simulink model "morrison"  (Simulink 7.8)
settings: Solver=ode45  StartTime=0.0  StopTime=2000.0  RelTol=1e-3
undefined symbols (not defined in the file or in its folder): inRate, shift
libraries: WaveformsLib x4, simulink x2
settings Model: Creator=Leo  LastModifiedBy=Leo

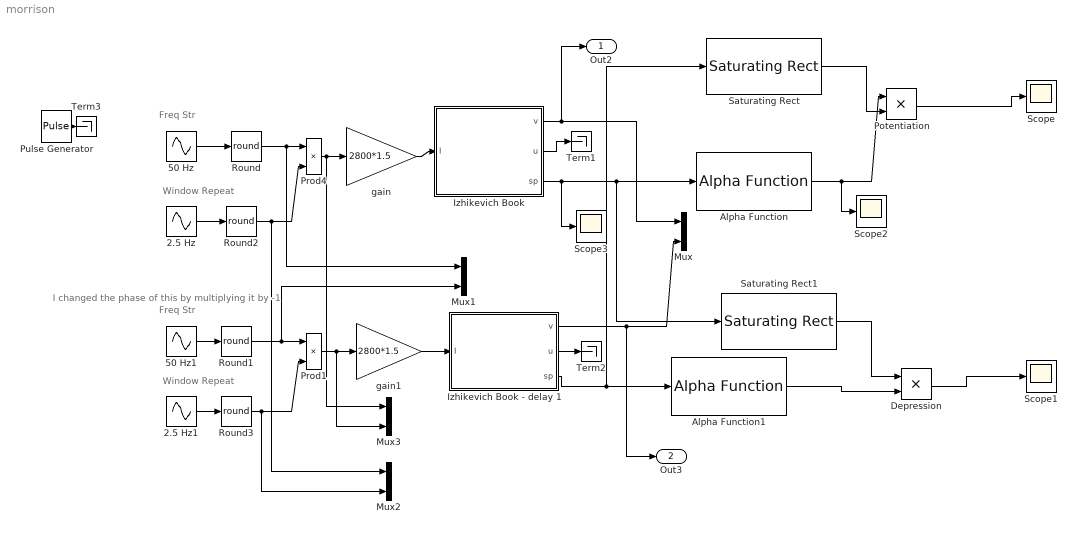
== system morrison ==
  note: Window Repeat
  note: Freq Str
  note: Window Repeat
  note: Freq Str
  note: I changed the phase of this by multiplying it by -1
  2.5 Hz : Sin  Amplitude=0.5  Bias=0.25  Frequency=2.5*2*pi/1000  Phase=pi  SampleTime=0
  2.5 Hz1 : Sin  Amplitude=0.5  Bias=0.25  Frequency=2.5*2*pi/1000  Phase=pi+shift*100/(2*pi*1000)  SampleTime=0
  50 Hz : Sin  Amplitude=0.5  Bias=inRate/20000  Frequency=inRate*2*pi/1000  Phase=-0*100/(2*pi*inRate)  SampleTime=0
  50 Hz1 : Sin  Amplitude=0.5  Bias=inRate/20000  Frequency=(inRate*2*pi)/1000  Phase=-shift*100/(2*pi*inRate)  SampleTime=0
  Alpha Function : WaveformsLib/Alpha Function  tauDecay=2  onsetStr=1
  Alpha Function1 : WaveformsLib/Alpha Function  tauDecay=2  onsetStr=1
  Depression : Product  RndMeth=Zero
  Izhikevich Book : Subsystem  AncestorBlock=CompartmentsLib/Izhikevich Book  mask{settings=UserDefined, A=0.03, B=-2, C=-50, D=100, CP=100, K=0.7, VR=-60, VT=-40, VP=35, V0=-60, U0=0}
      mask prompts: settings "Parameter Settings"; A "a, recovery u time constant"; B "b, dynamics parameter"; C "c,  reset value v"; D "d, reset shift u"; CP "Cp, capacitance"; VR "Vr, voltage rest"; VT "Vt, voltage threshold"; VP "Vpeak, voltage peak reset"; V0 "V0, initial v value"; U0 "U0, initial u value"
      mask help:
      | Model from Eugene Izhikevich's book "Dynamical Systems in Neuroscience"
      |     (Equations 8.5 & 8.6 on page 273)
      | 9 Paramters are reducable to 4-parameter model.
      |
      | Simulink Model Design: Jesse Palma
      mask Help:
      | Model from Eugene Izhikevich's book
      | <a href=http://www.izhikevich.org/publications/dsn/index.htm>"Dynamical Systems in Neuroscience"</a>
      | <br>(Equations 8.5 & 8.6 on page 273)<br>
      | 9 Paramters are reducable to 4-parameter model.
      | <br><br>
      | Simulink Model Design: Jesse Palma
      mask StyleString: popup(Regular-Spiking(p274-283)|Motor(p287)|UserDefined),edit,edit,edit,edit,edit,edit,edit,edit,edit,edit,edit
      mask CallbackString:
      | maskStr = get_param(gcb,'MaskValues');
      | if strcmp(maskStr{1},'Regular-Spiking(p274-283)')
      |    maskStr = get_param(gcb,'MaskValues');
      |    maskStr{2} = '0.03'; %A
      |    maskStr{3} = '-2';   %B
      |    maskStr{4} = '-50';  %C
      |    maskStr{5} = '100';  %D
      |    maskStr{6} = '100';  %CP
      |    maskStr{7} = '0.7';  %K
      |    maskStr{8} = '-60';  %VR
      |    maskStr{9} = '-40';  %VT
      |    maskStr{10} = '35';  %VP
      |    maskStr{11} = '-60'; %V0
      |    maskStr{12} = '0';   %U0
      |    set_param(gcb, 'MaskValues', maskStr);
      | end
      | if strcmp(maskStr{1},'Motor(p287)')
      |    maskStr = get_param(gcb,'MaskValues');
      |    maskStr{2} = '0.01'; %A
      |    maskStr{3} = '-0.25';%B
      |    maskStr{4} = '-40';  %C
      |    maskStr{5} = '90';   %D
      |    maskStr{6} = '30';   %CP
      |    maskStr{7} = '3';    %K
      |    maskStr{8} = '-55';  %VR
      |    maskStr{9} = '-42';  %VT
      |    maskStr{10} = '10';  %VP
      |    maskStr{11} = '-55'; %V0
      |    maskStr{12} = '0';   %U0
      |    set_param(gcb, 'MaskValues', maskStr);
      | end|maskStr = get_param(gcb,'MaskValues');
      | maskStr{1} = 'UserDefined';
      | set_param(gcb, 'MaskValues', maskStr);|maskStr = get_param(gcb,'MaskValues');
      | maskStr{1} = 'UserDefined';
      | set_param(gcb, 'MaskValues', maskStr);|maskStr = get_param(gcb,'MaskValues');
      | maskStr{1} = 'UserDefined';
      | set_param(gcb, 'MaskValues', maskStr);|maskStr = get_param(gcb,'MaskValues');
      | maskStr{1} = 'UserDefined';
      | set_param(gcb, 'MaskValues', maskStr);|maskStr = get_param(gcb,'MaskValues');
      | maskStr{1} = 'UserDefined';
      | set_param(gcb, 'MaskValues', maskStr);|maskStr = get_param(gcb,'MaskValues');
      | maskStr{1} = 'UserDefined';
      | set_param(gcb, 'MaskValues', maskStr);|maskStr = get_param(gcb,'MaskValues');
      | maskStr{1} = 'UserDefined';
      | set_param(gcb, 'MaskValues', maskStr);|maskStr = get_param(gcb,'MaskValues');
      | maskStr{1} = 'UserDefined';
      | set_param(gcb, 'MaskValues', maskStr);|maskStr = get_param(gcb,'MaskValues');
      | maskStr{1} = 'UserDefined';
      | set_param(gcb, 'MaskValues', maskStr);|maskStr = get_param(gcb,'MaskValues');
      | maskStr{1} = 'UserDefined';
      | set_param(gcb, 'MaskValues', maskStr);|maskStr = get_param(gcb,'MaskValues');
      | maskStr{1} = 'UserDefined';
      | set_param(gcb, 'MaskValues', maskStr);
      mask Display: image(imread('../Libs/icons/Izhik.jpg'),'center');
  Izhikevich Book - delay 1 : Subsystem  AncestorBlock=CompartmentsLib/Izhikevich Book  mask{settings=UserDefined, A=0.03, B=-2, C=-50, D=100, CP=100, K=0.7, VR=-60, VT=-40, VP=35, V0=-60, U0=0}
      mask prompts: settings "Parameter Settings"; A "a, recovery u time constant"; B "b, dynamics parameter"; C "c,  reset value v"; D "d, reset shift u"; CP "Cp, capacitance"; VR "Vr, voltage rest"; VT "Vt, voltage threshold"; VP "Vpeak, voltage peak reset"; V0 "V0, initial v value"; U0 "U0, initial u value"
      mask help:
      | Model from Eugene Izhikevich's book "Dynamical Systems in Neuroscience"
      |     (Equations 8.5 & 8.6 on page 273)
      | 9 Paramters are reducable to 4-parameter model.
      |
      | Simulink Model Design: Jesse Palma
      mask Help:
      | Model from Eugene Izhikevich's book
      | <a href=http://www.izhikevich.org/publications/dsn/index.htm>"Dynamical Systems in Neuroscience"</a>
      | <br>(Equations 8.5 & 8.6 on page 273)<br>
      | 9 Paramters are reducable to 4-parameter model.
      | <br><br>
      | Simulink Model Design: Jesse Palma
      mask StyleString: popup(Regular-Spiking(p274-283)|Motor(p287)|UserDefined),edit,edit,edit,edit,edit,edit,edit,edit,edit,edit,edit
      mask CallbackString:
      | maskStr = get_param(gcb,'MaskValues');
      | if strcmp(maskStr{1},'Regular-Spiking(p274-283)')
      |    maskStr = get_param(gcb,'MaskValues');
      |    maskStr{2} = '0.03'; %A
      |    maskStr{3} = '-2';   %B
      |    maskStr{4} = '-50';  %C
      |    maskStr{5} = '100';  %D
      |    maskStr{6} = '100';  %CP
      |    maskStr{7} = '0.7';  %K
      |    maskStr{8} = '-60';  %VR
      |    maskStr{9} = '-40';  %VT
      |    maskStr{10} = '35';  %VP
      |    maskStr{11} = '-60'; %V0
      |    maskStr{12} = '0';   %U0
      |    set_param(gcb, 'MaskValues', maskStr);
      | end
      | if strcmp(maskStr{1},'Motor(p287)')
      |    maskStr = get_param(gcb,'MaskValues');
      |    maskStr{2} = '0.01'; %A
      |    maskStr{3} = '-0.25';%B
      |    maskStr{4} = '-40';  %C
      |    maskStr{5} = '90';   %D
      |    maskStr{6} = '30';   %CP
      |    maskStr{7} = '3';    %K
      |    maskStr{8} = '-55';  %VR
      |    maskStr{9} = '-42';  %VT
      |    maskStr{10} = '10';  %VP
      |    maskStr{11} = '-55'; %V0
      |    maskStr{12} = '0';   %U0
      |    set_param(gcb, 'MaskValues', maskStr);
      | end|maskStr = get_param(gcb,'MaskValues');
      | maskStr{1} = 'UserDefined';
      | set_param(gcb, 'MaskValues', maskStr);|maskStr = get_param(gcb,'MaskValues');
      | maskStr{1} = 'UserDefined';
      | set_param(gcb, 'MaskValues', maskStr);|maskStr = get_param(gcb,'MaskValues');
      | maskStr{1} = 'UserDefined';
      | set_param(gcb, 'MaskValues', maskStr);|maskStr = get_param(gcb,'MaskValues');
      | maskStr{1} = 'UserDefined';
      | set_param(gcb, 'MaskValues', maskStr);|maskStr = get_param(gcb,'MaskValues');
      | maskStr{1} = 'UserDefined';
      | set_param(gcb, 'MaskValues', maskStr);|maskStr = get_param(gcb,'MaskValues');
      | maskStr{1} = 'UserDefined';
      | set_param(gcb, 'MaskValues', maskStr);|maskStr = get_param(gcb,'MaskValues');
      | maskStr{1} = 'UserDefined';
      | set_param(gcb, 'MaskValues', maskStr);|maskStr = get_param(gcb,'MaskValues');
      | maskStr{1} = 'UserDefined';
      | set_param(gcb, 'MaskValues', maskStr);|maskStr = get_param(gcb,'MaskValues');
      | maskStr{1} = 'UserDefined';
      | set_param(gcb, 'MaskValues', maskStr);|maskStr = get_param(gcb,'MaskValues');
      | maskStr{1} = 'UserDefined';
      | set_param(gcb, 'MaskValues', maskStr);|maskStr = get_param(gcb,'MaskValues');
      | maskStr{1} = 'UserDefined';
      | set_param(gcb, 'MaskValues', maskStr);
      mask Display: image(imread('../Libs/icons/Izhik.jpg'),'center');
  Mux{,1..3} (4 alike) : Mux  Inputs=2
  Potentiation : Product  RndMeth=Zero
  Prod1 : Product  RndMeth=Zero
  Prod4 : Product  RndMeth=Zero
  Pulse Generator : DiscretePulseGenerator  PulseType=Time based  Period=1000/inRate  PhaseDelay=shift/(inRate)+ shift*(1.12) + 49
  Round{,1..3} (4 alike) : Rounding  Operator=round
  Saturating Rect : WaveformsLib/Saturating Rect  squareWidth=1  squareHeight=1
  Saturating Rect1 : WaveformsLib/Saturating Rect  squareWidth=1  squareHeight=1
  Scope{,1..3} (4 alike) : Scope
      Scope2 settings: SaveName=ScopeData2
      Scope3 settings: SaveName=ScopeData3
  Term1 : Terminator
  Term2 : Terminator
  Term3 : Terminator
  gain : Gain  Gain=2800*1.5
  gain1 : Gain  Gain=2800*1.5
  Out2 : Outport
  Out3 : Outport  Port=2
  wires:
  gain/1 -> Izhikevich Book/1(I)
  Round/1 -> Prod4/1, Mux1/1
  50 Hz/1 -> Round/1
  Round2/1 -> Prod4/2, Mux2/1
  Prod4/1 -> gain/1, Mux3/1
  2.5 Hz/1 -> Round2/1
  gain1/1 -> Izhikevich Book - delay 1/1(I)
  Round1/1 -> Prod1/1, Mux1/2
  50 Hz1/1 -> Round1/1
  Round3/1 -> Prod1/2, Mux2/2
  Prod1/1 -> gain1/1, Mux3/2
  2.5 Hz1/1 -> Round3/1
  Izhikevich Book/1(v) -> Mux/1, Out2/1
  Izhikevich Book - delay 1/1(v) -> Out3/1, Mux/2
  Izhikevich Book - delay 1/3(sp) -> Alpha Function1/1, Saturating Rect/1
  Izhikevich Book/3(sp) -> Alpha Function/1, Saturating Rect1/1, Scope3/1
  Izhikevich Book/2(u) -> Term1/1
  Izhikevich Book - delay 1/2(u) -> Term2/1
  Pulse Generator/1 -> Term3/1
  Alpha Function/1 -> Potentiation/1, Scope2/1
  Potentiation/1 -> Scope/1
  Depression/1 -> Scope1/1
  Alpha Function1/1 -> Depression/2
  Saturating Rect/1 -> Potentiation/2
  Saturating Rect1/1 -> Depression/1

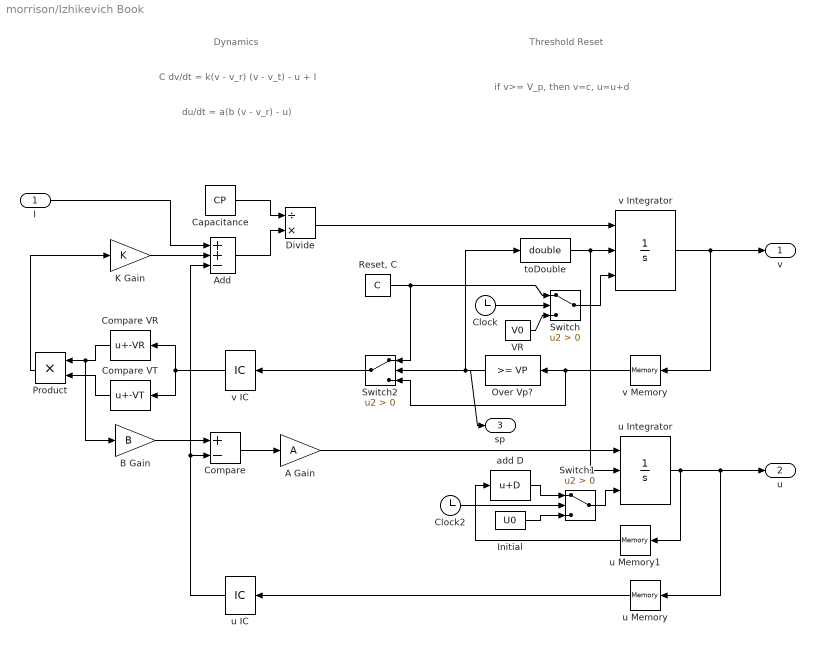
== system morrison/Izhikevich Book ==
  note: C dv/dt = k(v - v_r) (v - v_t) - u + I
  note: du/dt = a(b (v - v_r) - u)
  note: if v>= V_p, then
      | v=c, u=u+d
  note: Dynamics
  note: Threshold Reset
  I : Inport
  " Initial" : Constant  Value=U0
  A Gain : Gain  Gain=A
  Add : Sum  Inputs=++-
  B Gain : Gain  Gain=B
  Capacitance : Constant  Value=CP
  Clock : Clock
  Clock2 : Clock
  Compare : Sum  Inputs=+-
  Compare VR : Bias  Bias=-VR
  Compare VT : Bias  Bias=-VT
  Divide : Product  Inputs=/*
  K Gain : Gain  Gain=K
  Over Vp? : simulink/Logic and Bit Operations/Compare To Constant  relop=>=  const=VP  OutDataTypeStr=boolean  ZeroCross=off
  Product : Product  RndMeth=Zero
  "Reset, C" : Constant  Value=C
  Switch : Switch  Criteria=u2 > Threshold  ZeroCross=off
  Switch1 : Switch  Criteria=u2 > Threshold  ZeroCross=off
  Switch2 : Switch  Criteria=u2 > Threshold  ZeroCross=off
  VR : Constant  Value=V0
  add D : Bias  Bias=D
  toDouble : DataTypeConversion  OutDataTypeStr=double
  u IC : InitialCondition  Value=U0
  u Integrator : Integrator  ExternalReset=rising  InitialConditionSource=external  ZeroCross=off
  u Memory : Memory
  u Memory1 : Memory
  v IC : InitialCondition  Value=V0
  v Integrator : Integrator  ExternalReset=rising  InitialConditionSource=external  InitialCondition=VR  ZeroCross=off
  v Memory : Memory
  v : Outport
  u : Outport  Port=2
  sp : Outport  Port=3
  wires:
  u Memory1/1 -> add D/1
  VR/1 -> Switch/3
  Capacitance/1 -> Divide/1
  Add/1 -> Divide/2
  toDouble/1 -> v Integrator/2, u Integrator/2
  v Integrator/1 -> v/1, v Memory/1
  K Gain/1 -> Add/2
  Compare VT/1 -> Product/2
  Compare VR/1 -> B Gain/1, Product/1
  I/1 -> Add/1
  Product/1 -> K Gain/1
  u Memory/1 -> u IC/1
  B Gain/1 -> Compare/1
  Compare/1 -> A Gain/1
  v IC/1 -> Compare VT/1, Compare VR/1
  u IC/1 -> Add/3, Compare/2
  Switch/1 -> v Integrator/3
  Clock/1 -> Switch/2
  "Reset, C"/1 -> Switch2/1, Switch/1
  u Integrator/1 -> u Memory1/1, u/1, u Memory/1
  Divide/1 -> v Integrator/1
  A Gain/1 -> u Integrator/1
  Clock2/1 -> Switch1/2
  Switch1/1 -> u Integrator/3
  add D/1 -> Switch1/1
  " Initial"/1 -> Switch1/3
  Switch2/1 -> v IC/1
  v Memory/1 -> Switch2/3, Over Vp?/1
  Over Vp?/1 -> sp/1, Switch2/2, toDouble/1

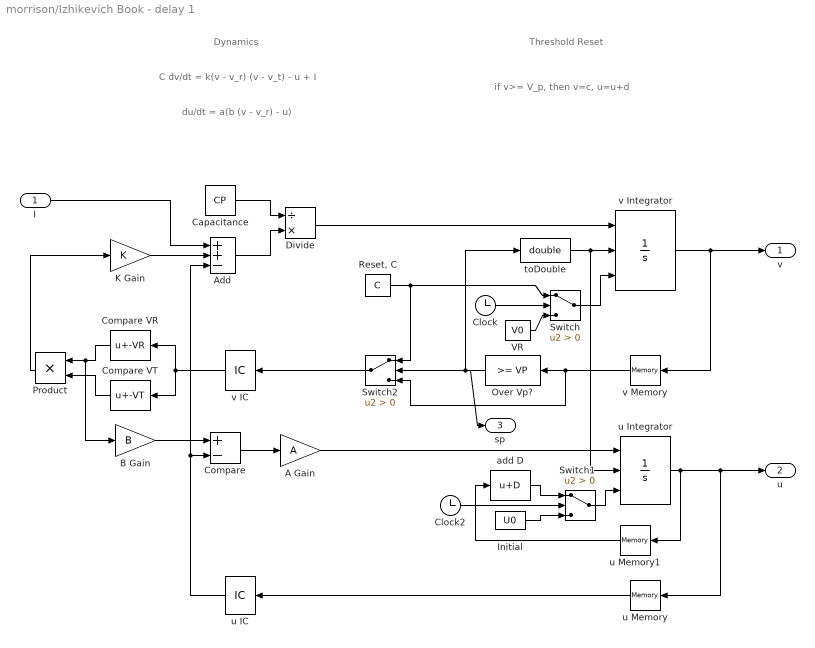
== system morrison/Izhikevich Book - delay 1 ==
  note: C dv/dt = k(v - v_r) (v - v_t) - u + I
  note: du/dt = a(b (v - v_r) - u)
  note: if v>= V_p, then
      | v=c, u=u+d
  note: Dynamics
  note: Threshold Reset
  I : Inport
  " Initial" : Constant  Value=U0
  A Gain : Gain  Gain=A
  Add : Sum  Inputs=++-
  B Gain : Gain  Gain=B
  Capacitance : Constant  Value=CP
  Clock : Clock
  Clock2 : Clock
  Compare : Sum  Inputs=+-
  Compare VR : Bias  Bias=-VR
  Compare VT : Bias  Bias=-VT
  Divide : Product  Inputs=/*
  K Gain : Gain  Gain=K
  Over Vp? : simulink/Logic and Bit Operations/Compare To Constant  relop=>=  const=VP  OutDataTypeStr=boolean  ZeroCross=off
  Product : Product  RndMeth=Zero
  "Reset, C" : Constant  Value=C
  Switch : Switch  Criteria=u2 > Threshold  ZeroCross=off
  Switch1 : Switch  Criteria=u2 > Threshold  ZeroCross=off
  Switch2 : Switch  Criteria=u2 > Threshold  ZeroCross=off
  VR : Constant  Value=V0
  add D : Bias  Bias=D
  toDouble : DataTypeConversion  OutDataTypeStr=double
  u IC : InitialCondition  Value=U0
  u Integrator : Integrator  ExternalReset=rising  InitialConditionSource=external  ZeroCross=off
  u Memory : Memory
  u Memory1 : Memory
  v IC : InitialCondition  Value=V0
  v Integrator : Integrator  ExternalReset=rising  InitialConditionSource=external  InitialCondition=VR  ZeroCross=off
  v Memory : Memory
  v : Outport
  u : Outport  Port=2
  sp : Outport  Port=3
  wires:
  u Memory1/1 -> add D/1
  VR/1 -> Switch/3
  Capacitance/1 -> Divide/1
  Add/1 -> Divide/2
  toDouble/1 -> v Integrator/2, u Integrator/2
  v Integrator/1 -> v/1, v Memory/1
  K Gain/1 -> Add/2
  Compare VT/1 -> Product/2
  Compare VR/1 -> B Gain/1, Product/1
  I/1 -> Add/1
  Product/1 -> K Gain/1
  u Memory/1 -> u IC/1
  B Gain/1 -> Compare/1
  Compare/1 -> A Gain/1
  v IC/1 -> Compare VT/1, Compare VR/1
  u IC/1 -> Add/3, Compare/2
  Switch/1 -> v Integrator/3
  Clock/1 -> Switch/2
  "Reset, C"/1 -> Switch2/1, Switch/1
  u Integrator/1 -> u Memory1/1, u/1, u Memory/1
  Divide/1 -> v Integrator/1
  A Gain/1 -> u Integrator/1
  Clock2/1 -> Switch1/2
  Switch1/1 -> u Integrator/3
  add D/1 -> Switch1/1
  " Initial"/1 -> Switch1/3
  Switch2/1 -> v IC/1
  v Memory/1 -> Switch2/3, Over Vp?/1
  Over Vp?/1 -> sp/1, Switch2/2, toDouble/1
